simulink model "P1_ADR"  (R2020b)
settings: Solver=VariableStepAuto  StartTime=0.0  StopTime=25  RelTol=1e-3
undefined symbols (not defined in the file): DiscIntNeverNeededParam
libraries: simulink x1
settings Model: Creator=marta  LastModifiedBy=marta

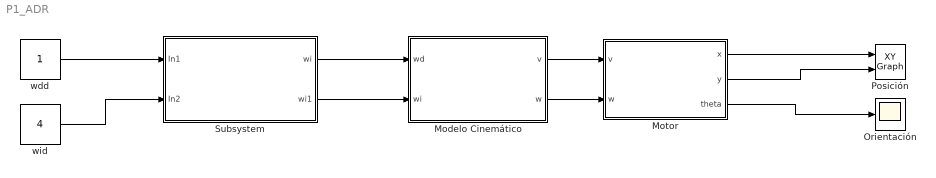
== system P1_ADR ==
  Modelo Cinemático : Subsystem
  Motor : Subsystem
  Orientación : Scope
  Posición : simulink/Sinks/XY Graph  xmin=-1  xmax=1  ymin=-1  ymax=1  st=-1
  Subsystem : Subsystem
  wdd : Constant  VectorParams1D=off  SampleTime=-1
  wid : Constant  Value=4  VectorParams1D=off  SampleTime=-1
  wires:
  Modelo Cinemático/1(v) -> Motor/1(v)
  Modelo Cinemático/2(w) -> Motor/2(w)
  Motor/1(x) -> Posición/1
  Motor/2(y) -> Posición/2
  Motor/3(theta) -> Orientación/1
  wdd/1 -> Subsystem/1(In1)
  Subsystem/1(wi) -> Modelo Cinemático/1(wd)
  Subsystem/2(wi1) -> Modelo Cinemático/2(wi)
  wid/1 -> Subsystem/2(In2)

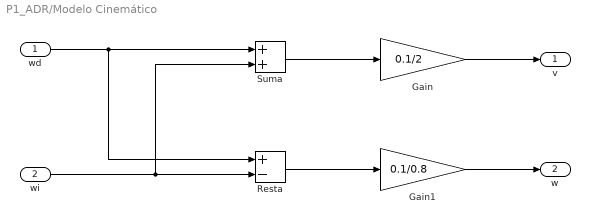
== system P1_ADR/Modelo Cinemático ==
  wd : Inport
  wi : Inport  Port=2
  Gain : Gain  Gain=0.1/2
  Gain1 : Gain  Gain=0.1/0.8
  Resta : Sum  Inputs=+-
  Suma : Sum
  v : Outport
  w : Outport  Port=2
  wires:
  wd/1 -> Resta/1, Suma/1
  Gain/1 -> v/1
  Suma/1 -> Gain/1
  wi/1 -> Resta/2, Suma/2
  Resta/1 -> Gain1/1
  Gain1/1 -> w/1

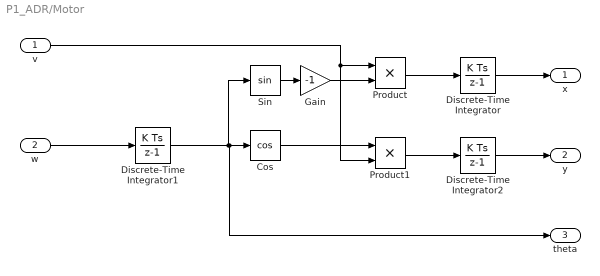
== system P1_ADR/Motor ==
  v : Inport
  w : Inport  Port=2
  Cos : Trigonometry  Operator=cos
  Discrete-Time Integrator : DiscreteIntegrator  SampleTime=-1  ICPrevOutput=DiscIntNeverNeededParam  ICPrevScaledInput=DiscIntNeverNeededParam
  Discrete-Time Integrator1 : DiscreteIntegrator  SampleTime=-1  ICPrevOutput=DiscIntNeverNeededParam  ICPrevScaledInput=DiscIntNeverNeededParam
  Discrete-Time Integrator2 : DiscreteIntegrator  SampleTime=-1  ICPrevOutput=DiscIntNeverNeededParam  ICPrevScaledInput=DiscIntNeverNeededParam
  Gain : Gain  Gain=-1
  Product : Product
  Product1 : Product
  Sin : Trigonometry
  x : Outport
  y : Outport  Port=2
  theta : Outport  Port=3
  wires:
  Gain/1 -> Product/2
  Product/1 -> Discrete-Time Integrator/1
  Sin/1 -> Gain/1
  v/1 -> Product1/2, Product/1
  Discrete-Time Integrator/1 -> x/1
  Discrete-Time Integrator1/1 -> Sin/1, theta/1, Cos/1
  Cos/1 -> Product1/1
  Product1/1 -> Discrete-Time Integrator2/1
  w/1 -> Discrete-Time Integrator1/1
  Discrete-Time Integrator2/1 -> y/1

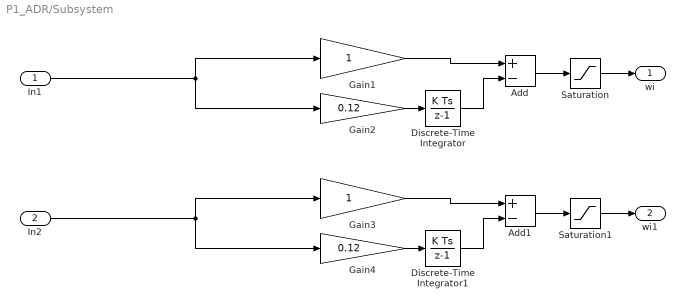
== system P1_ADR/Subsystem ==
  In1 : Inport
  In2 : Inport  Port=2
  Add : Sum  Inputs=+-
  Add1 : Sum  Inputs=+-
  Discrete-Time Integrator : DiscreteIntegrator  SampleTime=-1  ICPrevOutput=DiscIntNeverNeededParam  ICPrevScaledInput=DiscIntNeverNeededParam
  Discrete-Time Integrator1 : DiscreteIntegrator  SampleTime=-1  ICPrevOutput=DiscIntNeverNeededParam  ICPrevScaledInput=DiscIntNeverNeededParam
  Gain1 : Gain
  Gain2 : Gain  Gain=0.12
  Gain3 : Gain
  Gain4 : Gain  Gain=0.12
  Saturation : Saturate  UpperLimit=15  LowerLimit=-15
  Saturation1 : Saturate  UpperLimit=15  LowerLimit=-15
  wi : Outport
  wi1 : Outport  Port=2
  wires:
  In1/1 -> Gain2/1, Gain1/1
  Gain2/1 -> Discrete-Time Integrator/1
  Gain1/1 -> Add/1
  Add/1 -> Saturation/1
  Discrete-Time Integrator/1 -> Add/2
  In2/1 -> Gain4/1, Gain3/1
  Discrete-Time Integrator1/1 -> Add1/2
  Gain3/1 -> Add1/1
  Gain4/1 -> Discrete-Time Integrator1/1
  Saturation/1 -> wi/1
  Add1/1 -> Saturation1/1
  Saturation1/1 -> wi1/1
